simulink model "Regler_Kaskadierung_2"  (R2017b)
settings: Solver=FixedStepAuto  StartTime=0.0  StopTime=24000  FixedStep=0.5  RelTol=1e-3
values from neighbouring files (symbols this model uses):
  Kd_S = Kp_S*Tv_S    [Regler_Kaskadierung_2.m]    (also in Regler_Kaskadierung_2_editor.m)
  Ki_S = Kp_S/Tn_S    [Regler_Kaskadierung_2.m]    (also in Regler_Kaskadierung_2_editor.m)
  Kp_M = (0.35/K_Mantel)*(T1_Mantel/Tu)    (= 1.76744186047)    [Regler_Kaskadierung.m]    (also in Regler_Kaskadierung_2.m = 5; Regler_Kaskadierung_2_editor.m = 5; Regler_Mantel.m = (0.35/K_Mantel)*(T1_Mantel/Tu))
  Kp_S = (0.6*Tg_S)/(K_S*Tu_S)    [Regler_Kaskadierung_2.m]    (also in Regler_Kaskadierung_2_editor.m)
  Tt_S = sqrt(Tn_S*Tv_S)    [Regler_Kaskadierung_2.m]    (also in Regler_Kaskadierung_2_editor.m)
libraries: cstblocks x2
settings Model: Creator=arbno  LastModifiedBy=arbno

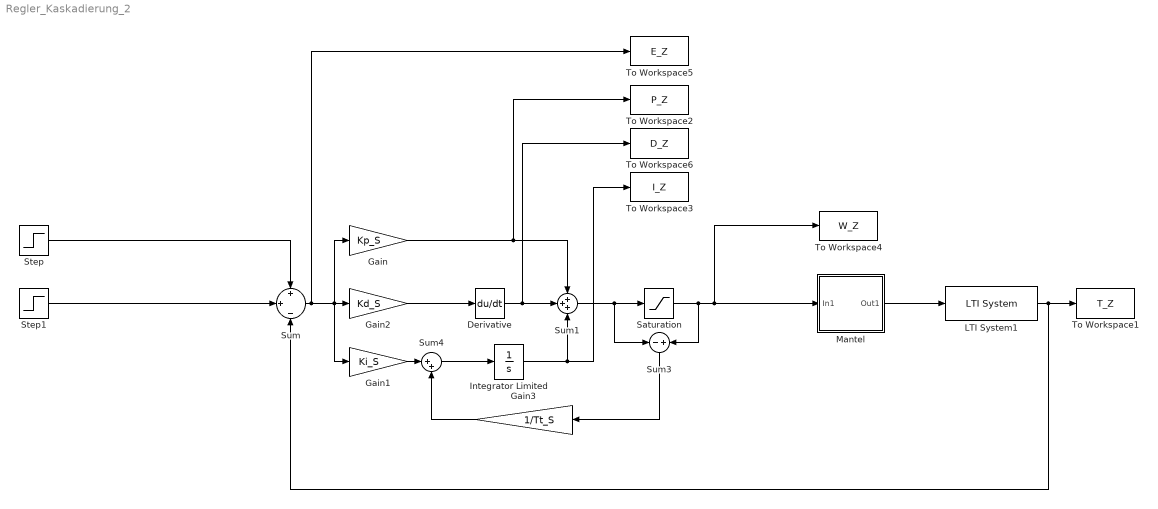
== system Regler_Kaskadierung_2 ==
  Derivative : Derivative
  Gain : Gain  Gain=Kp_S
  Gain1 : Gain  Gain=Ki_S
  Gain2 : Gain  Gain=Kd_S
  Gain3 : Gain  Gain=1/Tt_S
  Integrator Limited : Integrator  UpperSaturationLimit=150  LowerSaturationLimit=-150
  LTI System1 : cstblocks/LTI System  sys=G_Zelle  IC=[]
  Mantel : Subsystem
  Saturation : Saturate  UpperLimit=141  LowerLimit=0
  Step : Step  Time=0  After=80  SampleTime=0
  Step1 : Step  Time=0  After=0  SampleTime=0
  Sum : Sum  Inputs=+|+|-
  Sum1 : Sum  Inputs=+++
  Sum3 : Sum  Inputs=-|+
  Sum4 : Sum  Inputs=|++
  To Workspace1 : ToWorkspace  VariableName=T_Z  SaveFormat=Structure With Time  SampleTime=-1
  To Workspace2 : ToWorkspace  VariableName=P_Z  SaveFormat=Structure With Time  SampleTime=-1
  To Workspace3 : ToWorkspace  VariableName=I_Z  SaveFormat=Structure With Time  SampleTime=-1
  To Workspace4 : ToWorkspace  VariableName=W_Z  SaveFormat=Structure With Time  SampleTime=-1
  To Workspace5 : ToWorkspace  VariableName=E_Z  SaveFormat=Structure With Time  SampleTime=-1
  To Workspace6 : ToWorkspace  VariableName=D_Z  SaveFormat=Structure With Time  SampleTime=-1
  wires:
  Mantel/1(Out1) -> LTI System1/1
  Gain2/1 -> Derivative/1
  LTI System1/1 -> To Workspace1/1, Sum/3
  Sum1/1 -> Sum3/1, Saturation/1
  Step/1 -> Sum/1
  Derivative/1 -> To Workspace6/1, Sum1/2
  Sum4/1 -> Integrator Limited/1
  Sum/1 -> To Workspace5/1, Gain1/1, Gain2/1, Gain/1
  Gain/1 -> Sum1/1, To Workspace2/1
  Saturation/1 -> Sum3/2, Mantel/1(In1), To Workspace4/1
  Integrator Limited/1 -> To Workspace3/1, Sum1/3
  Sum3/1 -> Gain3/1
  Gain1/1 -> Sum4/1
  Gain3/1 -> Sum4/2
  Step1/1 -> Sum/2

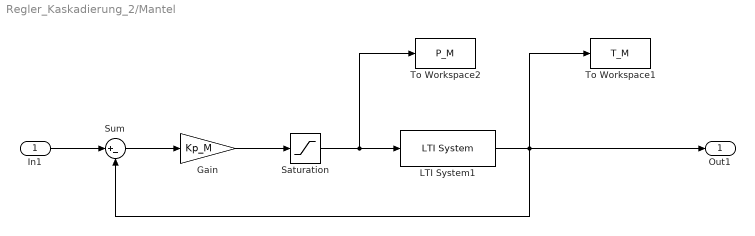
== system Regler_Kaskadierung_2/Mantel ==
  In1 : Inport
  Gain : Gain  Gain=Kp_M
  LTI System1 : cstblocks/LTI System  sys=G_Mantel  IC=[]
  Saturation : Saturate  UpperLimit=1  LowerLimit=0
  Sum : Sum  Inputs=|+-
  To Workspace1 : ToWorkspace  VariableName=T_M  SaveFormat=Structure With Time  SampleTime=-1
  To Workspace2 : ToWorkspace  VariableName=P_M  SaveFormat=Structure With Time  SampleTime=-1
  Out1 : Outport
  wires:
  LTI System1/1 -> Out1/1, Sum/2, To Workspace1/1
  Sum/1 -> Gain/1
  In1/1 -> Sum/1
  Saturation/1 -> To Workspace2/1, LTI System1/1
  Gain/1 -> Saturation/1
